simulink model "TestBed_simulation"  (R2024b)
settings: Solver=VariableStepAuto  StartTime=0.0  StopTime=1  RelTol=1e-3  AbsTol=1e-3
libraries: spsThreePhaseVIMeasurementLib x4, spsThreePhasePISectionLineLib x3, spsThreePhaseBreakerLib x2, spsThreePhaseParallelRLCLoadLib x1, spsThreePhaseProgrammableVoltageSourceLib x1, spsThreePhaseSeriesRLCBranchLib x1, spsWindTurbineInductionGeneratorPhasorTypeLib x1, sps_lib x1
settings Model: Creator=root  LastModifiedBy=keert
settings SolverCC: AutoScaleAbsTol=off  AlgebraicLoopSolver=TrustRegion  MaxZcPerStep=1
settings DebuggingCC: UnconnectedInputMsg=warning  UnconnectedOutputMsg=warning  UnconnectedLineMsg=warning  SymbolicDimsDataTypeCodeGenerationDiagnostic=none
settings ModelReferenceCC: EnableRefExpFcnMdlSchedulingChecks=on
settings SFSimCC: CustomCodeUndefinedFunction=UseInterfaceOnly
settings RTWCC: GPUComputeCapability=3.5  DLArmComputeVersion=19.05
settings SimscapeCC: SimscapeLogType=all  SimscapeLogSimulationStatistics=on  SimscapeLogDataHistory=10000

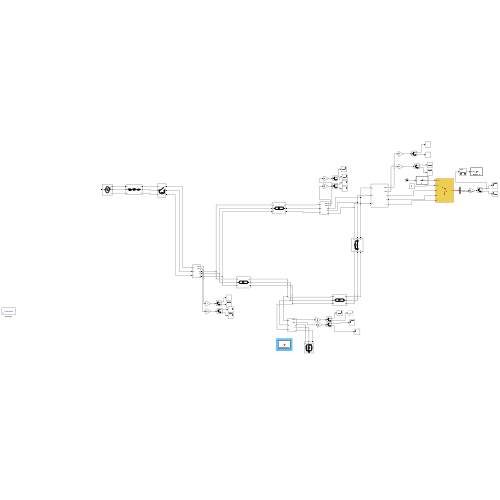
[thumbnail: Simulink's stored preview of the top-level diagram]
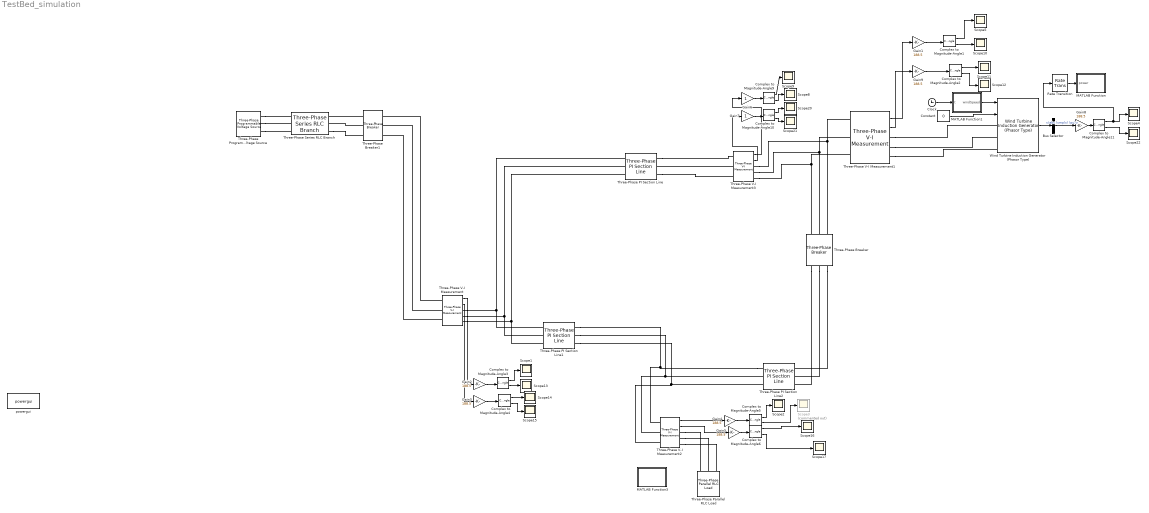
== system TestBed_simulation ==
  Bus Selector : BusSelector  OutputSignals=Iabc (cmplx) (pu)
  Clock : Clock
  Complex to Magnitude-Angle{1..6,9..11} (9 alike) : ComplexToMagnitudeAngle
  Constant : Constant  Value=0
  Gain{1..5,8..9} (7 alike) : Gain  Gain=188.5
  Gain6 : Gain
  Gain7 : Gain
  MATLAB Function : MATLAB Function  TreatAsAtomicUnit=on
  MATLAB Function1 : MATLAB Function  TreatAsAtomicUnit=on
  MATLAB Function3 : MATLAB Function  TreatAsAtomicUnit=on
  Rate Transition : RateTransition  OutPortSampleTime=0.01
  Scope{1..2,4..5,8..17,20..22} (17 alike) : Scope
  Scope3 : Scope  Commented=on
  Three-Phase PI Section Line : spsThreePhasePISectionLineLib/Three-Phase PI Section Line  LConnTagsString=a|b|c  RConnTagsString=A|B|C  Length=100  Frequency=60  Resistances=[ 0.01273 0.3864]  Inductances="[ 0.9337e-3  4.1264e-3]"  Capacitances=[12.74e-9 7.751e-9]
  Three-Phase PI Section Line1 : spsThreePhasePISectionLineLib/Three-Phase PI Section Line  LConnTagsString=a|b|c  RConnTagsString=A|B|C  Length=100  Frequency=60  Resistances=[ 0.01273 0.3864]  Inductances="[ 0.9337e-3  4.1264e-3]"  Capacitances=[12.74e-9 7.751e-9]
  Three-Phase PI Section Line2 : spsThreePhasePISectionLineLib/Three-Phase PI Section Line  LConnTagsString=a|b|c  RConnTagsString=A|B|C  Length=100  Frequency=60  Resistances=[ 0.01273 0.3864]  Inductances="[ 0.9337e-3  4.1264e-3]"  Capacitances=[12.74e-9 7.751e-9]
  Three-Phase Parallel RLC Load : spsThreePhaseParallelRLCLoadLib/Three-Phase Parallel RLC Load  LConnTagsString=A|B|C  Configuration=Y (grounded)  NominalVoltage=1000  Vabc=[1e3 1e3 1e3]  Vabcp=[1e3 1e3 1e3]  NominalFrequency=60  UnbalancedPower=off  ActivePower=P_Load  InductivePower=100  CapacitivePower=100  Pabc=[10e3 9e3 11e3]  QLabc=[100 90 110]  QCabc=[100 90 110]  Pabcp=[10e3 9e3 11e3]  QLabcp=[100 90 110]  QCabcp=[100 90 110]  Measurements=None  LoadType=constant Z
  Three-Phase Programmable Voltage Source : spsThreePhaseProgrammableVoltageSourceLib/Three-Phase Programmable Voltage Source  PositiveSequence="[230000  0 50]"  VariationEntity=None  VariationType=Table of time-amplitude pairs  VariationTypeAlt=Step  VariationStep=0.5  VariationRate=10  VariationMagnitude=0.3  VariationFrequency=2  VariationTiming=[1 2]  VariationPhaseA=off  Amplitudes=[1 0.8 1.2 1.0]  TimeValues=[0 0.1 0.15 0.2]  HarmonicGeneration=off  HarmonicA=[3 0.2 -25 0]  HarmonicB=[2 0.15 35 2]  Timing="[0.05  3]"  BusType=swing  Pref=0  Qref=0  Qmin=-inf  Qmax=inf
  Three-Phase Series RLC Branch : spsThreePhaseSeriesRLCBranchLib/Three-Phase Series RLC Branch  LConnTagsString=A|B|C  RConnTagsString=A|B|C  BranchType=RLC  Resistance=0.1  Inductance=0.0006  Capacitance=0  Measurements=None
  Three-Phase V-I Measurement{,1..3} (4 alike) : spsThreePhaseVIMeasurementLib/Three-Phase V-I Measurement  VoltageMeasurement=phase-to-ground  SetLabelV=off  LabelV=Vabc  Vpu=off  VpuLL=off  CurrentMeasurement=yes  SetLabelI=off  LabelI=Iabc  Ipu=off  Pbase=100e6  Vbase=500e3  OutputType=Complex  PhasorSimulation=off  PSBequivalent=0
  Three-Phase Breaker : spsThreePhaseBreakerLib/Three-Phase Breaker  InitialState=closed  SwitchA=on  SwitchB=on  SwitchC=on  SwitchTimes="[2/60  3/60]"  External=off  BreakerResistance=0.01  SnubberResistance=1e6  SnubberCapacitance=inf  Measurements=None
  Three-Phase Breaker1 : spsThreePhaseBreakerLib/Three-Phase Breaker  InitialState=open  SwitchA=on  SwitchB=on  SwitchC=on  SwitchTimes="[1/60  5/60]"  External=off  BreakerResistance=0.01  SnubberResistance=1e6  SnubberCapacitance=inf  Measurements=None
  Wind Turbine Induction Generator (Phasor Type) : spsWindTurbineInductionGeneratorPhasorTypeLib/Wind Turbine Induction Generator (Phasor Type)  ExternalTm=off  nom=[1.5e6/0.9, 575, 60]  sta=[ 0.004843, 0.1248]  rot=[ 0.004377, 0.1791]  Lm=6.77  mec=[5.04, 0.01, 3]  init="[ -0.01,0,   0,0,0,   0,0,0 ]"  pitch_angle=0  Pmec=1.5e6  wind_base=9  speed_nom=1  P_wind_base=1  K_pitch_gain=[5 25]  pitch_max=45  pitch_rate=2
      settings: LibrarySourceBlock=|
      | sps_lib/Electrical Machines/Wind Turbine
      | Induction Generator
      | (Phasor Type)
  powergui : sps_lib/powergui  Priority=1  SimulationMode=Continuous  SampleTime=50e-6  frequency=60  Iterations=50  frequencyindice=50  Pbase=100e6  ErrMax=1e-4  UnitsV=kV  UnitsW=MW  buscounter=0  FunctionMessages=off  echomessages=off  EnableUseOfTLC=off  CurrentSourceSwitches=off  DisableSnubberDevices=off  DisableRonSwitches=off  DisableVfSwitches=off  DisplayEquations=off  AutomaticDiscreteSolvers=off  SolverType=Tustin/Backward Euler (TBE)  Interpol=off  ExternalGateDelay=off  methode=off  Ts=100  x0status=blocks  SPID=on  SwTol=0  HookPort=off  NonlinearTolerance=1e-4  nMaxIteration=100  ContinueOnMaxIteration=off  RestoreLinks=warning  ResistiveCurrentMeasurement=off  Frange=[0:2:500]  Ylog=off  Xlog=on  ShowGrid=off  save=off  variable=ZData  structure=0  ZoomFFT=off  StartTime=0.0  cycles=1  DisplayStyle=1  fundamental=60  FreqAxis=off  MaxFrequency=1000  frequencyindicesteady=1  RmsSteady=1  display=off
  wires:
  Three-Phase V-I Measurement2/1 -> Gain4/1
  Three-Phase V-I Measurement2/2 -> Gain5/1
  Three-Phase V-I Measurement/1 -> Gain2/1
  Three-Phase V-I Measurement/2 -> Gain3/1
  Gain2/1 -> Complex to Magnitude-Angle3/1
  Gain3/1 -> Complex to Magnitude-Angle4/1
  Complex to Magnitude-Angle3/1 -> Scope1/1
  Complex to Magnitude-Angle3/2 -> Scope13/1
  Complex to Magnitude-Angle4/1 -> Scope14/1
  Complex to Magnitude-Angle4/2 -> Scope15/1
  Gain5/1 -> Complex to Magnitude-Angle6/1
  Gain4/1 -> Complex to Magnitude-Angle5/1
  Complex to Magnitude-Angle5/1 -> Scope2/1
  Complex to Magnitude-Angle5/2 -> Scope3/1
  Complex to Magnitude-Angle6/1 -> Scope16/1
  Complex to Magnitude-Angle6/2 -> Scope17/1
  Three-Phase V-I Measurement3/1 -> Gain6/1
  Three-Phase V-I Measurement3/2 -> Gain7/1
  Gain6/1 -> Complex to Magnitude-Angle9/1
  Gain7/1 -> Complex to Magnitude-Angle10/1
  Complex to Magnitude-Angle9/1 -> Scope9/1
  Complex to Magnitude-Angle9/2 -> Scope8/1
  Complex to Magnitude-Angle10/1 -> Scope20/1
  Complex to Magnitude-Angle10/2 -> Scope21/1
  Gain8/1 -> Complex to Magnitude-Angle11/1
  Complex to Magnitude-Angle11/2 -> Scope22/1
  Bus Selector/1 -> Gain8/1  "<Iabc (cmplx) (pu)>"
  Three-Phase V-I Measurement1/1 -> Gain1/1
  Three-Phase V-I Measurement1/2 -> Gain9/1
  Gain1/1 -> Complex to Magnitude-Angle1/1
  Gain9/1 -> Complex to Magnitude-Angle2/1
  Complex to Magnitude-Angle1/2 -> Scope10/1
  Complex to Magnitude-Angle2/1 -> Scope11/1
  Complex to Magnitude-Angle2/2 -> Scope12/1
  Complex to Magnitude-Angle1/1 -> Scope5/1
  Wind Turbine Induction Generator (Phasor Type)/1 -> Bus Selector/1
  Complex to Magnitude-Angle11/1 -> Rate Transition/1, Scope4/1
  Rate Transition/1 -> MATLAB Function/1(power)
  MATLAB Function1/1(windSpeed) -> Wind Turbine Induction Generator (Phasor Type)/1
  Clock/1 -> MATLAB Function1/1(t)
  Constant/1 -> Wind Turbine Induction Generator (Phasor Type)/2
  connections:
  Three-Phase Programmable Voltage Source/RConn1 -- Three-Phase Series RLC Branch/LConn1
  Three-Phase Programmable Voltage Source/RConn2 -- Three-Phase Series RLC Branch/LConn2
  Three-Phase Programmable Voltage Source/RConn3 -- Three-Phase Series RLC Branch/LConn3
  Three-Phase Breaker1/LConn1 -- Three-Phase Series RLC Branch/RConn1
  Three-Phase Breaker1/LConn2 -- Three-Phase Series RLC Branch/RConn2
  Three-Phase Series RLC Branch/RConn3 -- Three-Phase Breaker1/LConn3
  Three-Phase PI Section Line1/LConn1 -- Three-Phase PI Section Line/LConn1 -- Three-Phase V-I Measurement/RConn1
  Three-Phase PI Section Line1/RConn2 -- Three-Phase PI Section Line2/LConn2 -- Three-Phase V-I Measurement2/LConn2
  Three-Phase Breaker/RConn3 -- Three-Phase PI Section Line2/RConn3
  Three-Phase Breaker/RConn2 -- Three-Phase PI Section Line2/RConn2
  Three-Phase Breaker/RConn1 -- Three-Phase PI Section Line2/RConn1
  Three-Phase V-I Measurement3/LConn2 -- Three-Phase PI Section Line/RConn2
  Three-Phase Breaker/LConn1 -- Three-Phase V-I Measurement1/LConn1 -- Three-Phase V-I Measurement3/RConn1
  Three-Phase Breaker/LConn2 -- Three-Phase V-I Measurement1/LConn2 -- Three-Phase V-I Measurement3/RConn2
  Three-Phase Breaker/LConn3 -- Three-Phase V-I Measurement1/LConn3 -- Three-Phase V-I Measurement3/RConn3
  Three-Phase PI Section Line1/LConn2 -- Three-Phase PI Section Line/LConn2 -- Three-Phase V-I Measurement/RConn2
  Three-Phase PI Section Line1/LConn3 -- Three-Phase V-I Measurement/RConn3 -- Three-Phase PI Section Line/LConn3
  Three-Phase V-I Measurement/LConn1 -- Three-Phase Breaker1/RConn1
  Three-Phase V-I Measurement/LConn2 -- Three-Phase Breaker1/RConn2
  Three-Phase V-I Measurement/LConn3 -- Three-Phase Breaker1/RConn3
  Three-Phase PI Section Line/RConn1 -- Three-Phase V-I Measurement3/LConn1
  Three-Phase PI Section Line/RConn3 -- Three-Phase V-I Measurement3/LConn3
  Three-Phase V-I Measurement2/LConn1 -- Three-Phase PI Section Line2/LConn1 -- Three-Phase PI Section Line1/RConn1
  Three-Phase V-I Measurement2/LConn3 -- Three-Phase PI Section Line2/LConn3 -- Three-Phase PI Section Line1/RConn3
  Three-Phase V-I Measurement2/RConn1 -- Three-Phase Parallel RLC Load/LConn1
  Three-Phase V-I Measurement2/RConn2 -- Three-Phase Parallel RLC Load/LConn2
  Three-Phase V-I Measurement2/RConn3 -- Three-Phase Parallel RLC Load/LConn3
  Three-Phase V-I Measurement1/RConn1 -- Wind Turbine Induction Generator (Phasor Type)/LConn1
  Three-Phase V-I Measurement1/RConn2 -- Wind Turbine Induction Generator (Phasor Type)/LConn2
  Three-Phase V-I Measurement1/RConn3 -- Wind Turbine Induction Generator (Phasor Type)/LConn3

== matlab function TestBed_simulation/MATLAB Function ==
  data: power input
function writePipe(power)
    coder.extrinsic('sprintf', 'disp', 'sendToPipe');
    message = sprintf('Wind Power generated: %.3f', power(1));  % Use first element if array
    disp(message);
    sendToPipe(power(1));  % Send scalar value only
end

== matlab function TestBed_simulation/MATLAB Function3 ==
function updateLoad()
persistent previousInstruction

if isempty(previousInstruction)
    previousInstruction = blanks(10);
end

fid = fopen('\\wsl.localhost\Ubuntu\tmp\control_data_debug.txt', 'r');

if fid <= 0 
    disp("govinda");
    return;
end

instr = fgetl(fid);
fclose(fid);

if isempty(instr)
    return;
end

instr_padded = blanks(10);
instr_padded(1:length(instr)) = instr;

if ~strcmp(instr_padded, previousInstruction)
    

    if strcmp(instr, 'z')
        assignin('base', 'P_Load', 1000); % 100% of P_Load
        disp(instr);
    elseif strcmp(instr, 'y')
        assignin('base', 'P_Load', 750); % 75% of P_Load
        disp(instr);
    elseif strcmp(instr, 'x')
        assignin('base', 'P_Load', 500); % 50% of P_Load
        disp(instr);
    end

    previousInstruction = instr_padded;
end
end

== matlab function TestBed_simulation/MATLAB Function1 ==
  settings: updateMethod=DISCRETE
  data: t input; windSpeed output
function windSpeed = fcn(t)
% Generates smooth random wind speed based on current simulation time

persistent windHistory timeHistory

if isempty(windHistory)
    windHistory = 8 + 0.2 * randn(1, 1);
    timeHistory = t;
else
    deltaWind = 0.05 * randn();
    newWind = windHistory(end) + deltaWind;
    newWind = max(min(newWind, 15), 5);
    windHistory(end+1) = newWind;
    timeHistory(end+1) = t;
end

% Smoothing using a moving average
smoothWindow = 5;
if length(windHistory) >= smoothWindow
    windSpeed = mean(windHistory(end-smoothWindow+1:end));
else
    windSpeed = mean(windHistory);
end
fprintf('Time: %.2f s, Wind Speed: %.2f m/s\n', t, windSpeed);
